simulink library "VehiculeHypothese"  (R2018a)
settings: Solver=VariableStepAuto  StartTime=0.0  StopTime=10.0  RelTol=1e-3
settings Model: Creator=thomas.moser  LastModifiedBy=thomas.moser

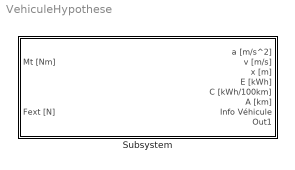
== system VehiculeHypothese ==
  Subsystem : Subsystem  mask{m=2250, mp=80, rr=0.33, s=1, cx=0.5, crr=0.015, mlimit=660, alimit=3, r=9.73, nr=0.9, nm=0.89, nc=0.89, cb=98}
      mask prompts: m "Poids [kg] :"; mp "Poids passagers [kg] :"; rr "Rayon de la roue [m] :"; s "Surface frontale [m^2] :"; cx "Coefficient de trainée [-] :"; crr "Coefficient de résistance aux roulements [-] :"; mlimit "Couple limite [Nm] :"; alimit "Accélération maximum [m/s^2] :"; r "Rapport de réduction [-] :"; nr "Rendement du réducteur [-] :"; nm "Rendement du moteur [-] :"; nc "Rendement du convertisseur [-] :"; cb "Capacité de la batterie [kWh] :"
      mask DialogControl Voiture Prompt: Voiture
      mask DialogControl Transmission Prompt: Bloc moteur
      mask DialogControl Electronique Prompt: Electronique
      mask Display: image('C:\Users\thomas.moser\Desktop\Capture24434.PNG');

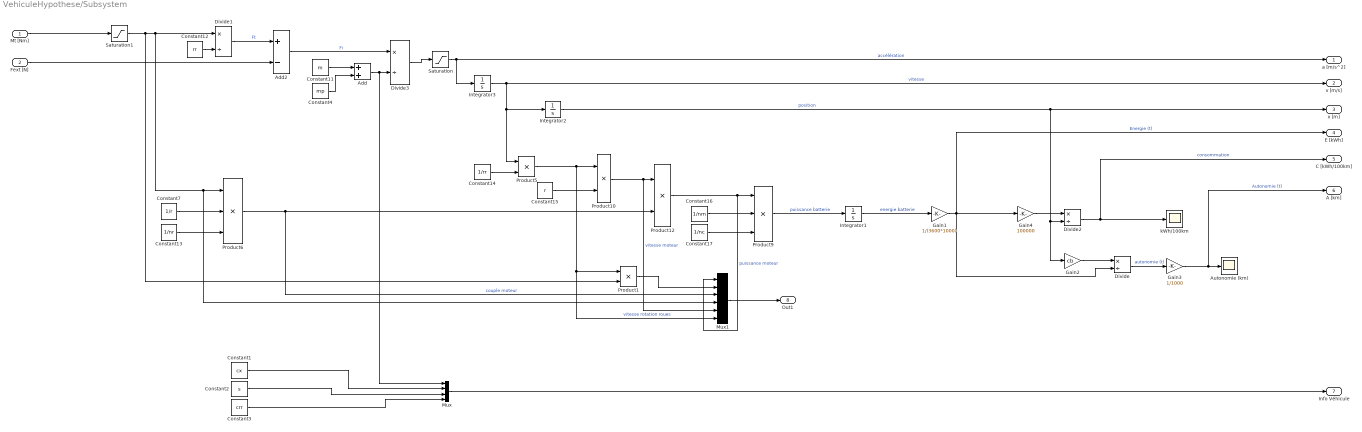
== system VehiculeHypothese/Subsystem ==
  Mt [Nm] : Inport
  Fext [N] : Inport  Port=2
  Add : Sum
  Add2 : Sum  Inputs=+-
  Autonomie (km) : Scope
  Constant1 : Constant  Value=cx
  Constant11 : Constant  Value=m
  Constant12 : Constant  Value=rr
  Constant13 : Constant  Value=1/nr
  Constant14 : Constant  Value=1/rr
  Constant15 : Constant  Value=r
  Constant16 : Constant  Value=1/nm
  Constant17 : Constant  Value=1/nc
  Constant2 : Constant  Value=s
  Constant3 : Constant  Value=crr
  Constant4 : Constant  Value=mp
  Constant7 : Constant  Value=1/r
  Divide{,1..3} (4 alike) : Product  Inputs=*/
  Gain1 : Gain  Gain=1/(3600*1000)
  Gain2 : Gain  Gain=cb
  Gain3 : Gain  Gain=1/1000
  Gain4 : Gain  Gain=100000
  Integrator1 : Integrator
  Integrator2 : Integrator
  Integrator3 : Integrator
  Mux : Mux
  Mux1 : Mux  Inputs=6
  Product{1,5,10,12} (4 alike) : Product
  Product6 : Product  Inputs=3
  Product9 : Product  Inputs=3
  Saturation : Saturate  UpperLimit=alimit  LowerLimit=-alimit
  Saturation1 : Saturate  UpperLimit=mlimit*r*nr  LowerLimit=-mlimit*r*nr
  "kWh/100km " : Scope
  a [m/s^2] : Outport
  v [m/s] : Outport  Port=2
  x [m] : Outport  Port=3
  E [kWh] : Outport  Port=4
  C [kWh/100km] : Outport  Port=5
  A [km] : Outport  Port=6
  Info Véhicule : Outport  Port=7
  Out1 : Outport  Port=8
  wires:
  Gain3/1 -> A [km]/1, Autonomie (km)/1  "Autonomie (t)"
  Constant14/1 -> Product5/2
  Product12/1 -> Mux1/1, Product9/1  "puissance moteur"
  Integrator3/1 -> v [m/s]/1, Integrator2/1, Product5/1  "vitesse"
  Constant12/1 -> Divide1/2
  Gain1/1 -> E [kWh]/1, Divide/2, Gain4/1  "Energie (t)"
  Saturation1/1 -> Product1/2, Divide1/1, Mux1/4, Product6/1
  Add2/1 -> Divide3/1  "Fi"
  Constant17/1 -> Product9/3
  Mt [Nm]/1 -> Saturation1/1
  Saturation/1 -> a [m/s^2]/1, Integrator3/1  "accélération"
  Divide3/1 -> Saturation/1
  Product5/1 -> Mux1/6, Product1/1, Product10/1  "vitesse rotation roues"
  Constant15/1 -> Product10/2
  Constant16/1 -> Product9/2
  Integrator2/1 -> x [m]/1, Gain2/1, Divide2/2  "position"
  Gain4/1 -> Divide2/1
  Product9/1 -> Integrator1/1  "puissance batterie"
  Constant13/1 -> Product6/3
  Divide1/1 -> Add2/1  "Ft"
  Constant7/1 -> Product6/2
  Divide2/1 -> C [kWh/100km]/1, "kWh/100km "/1  "consommation"
  Divide/1 -> Gain3/1  "autonomie (t)"
  Product6/1 -> Mux1/3, Product12/2  "couple moteur"
  Gain2/1 -> Divide/1
  Product10/1 -> Mux1/5, Product12/1  "vitesse moteur"
  Fext [N]/1 -> Add2/2
  Constant1/1 -> Mux/2
  Constant2/1 -> Mux/3
  Constant3/1 -> Mux/4
  Mux/1 -> Info Véhicule/1
  Constant4/1 -> Add/2
  Constant11/1 -> Add/1
  Add/1 -> Mux/1, Divide3/2
  Integrator1/1 -> Gain1/1  "energie batterie"
  Mux1/1 -> Out1/1
  Product1/1 -> Mux1/2
